simulink model "SSBaudio"  (R2015b)
settings: Solver=VariableStepAuto  StartTime=0.0  StopTime=10.0  RelTol=1e-3
undefined symbols (not defined in the file): SF_Frame, SF_PSF_SampPerSym, SF_Rsymbol
libraries: simrfV2util1 x4, dspxfrm3 x2, simrfV2elements x2, commanapbnd3 x2, commrflib2 x1, simrfV2sources1 x1, dspvision x1, commfilt2 x1
settings Model: Creator=dominikguz  LastModifiedBy=dominikguz

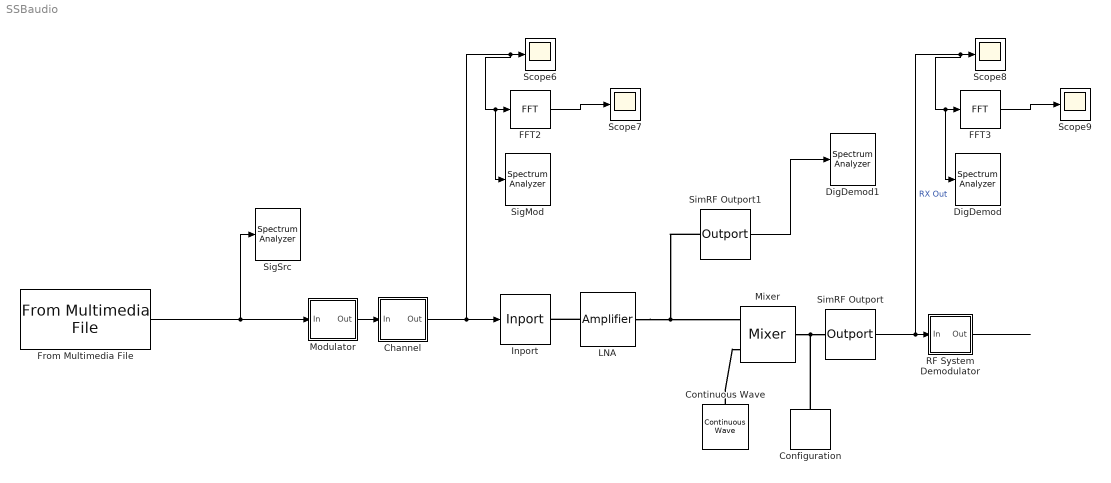
== system SSBaudio ==
  Channel : Subsystem
  Configuration : simrfV2util1/Configuration  AutoFreq=off  Tones="[5e8, 1.6e9]  Hz"  Harmonics=1  NormalizeCarrierPower=on  SolverType=Auto  StepSize=1/(SF_PSF_SampPerSym*SF_Rsymbol) s  AddNoise=on  Temperature=290.0 K  SolverDelFlag=0
  Continuous Wave : simrfV2sources1/Continuous Wave  CWSourceType=Ideal voltage  Z0=0  IVoltage=1 V  ICurrent=0 A  MagPower=0 W  QVoltage=0 V  QCurrent=0 A  AnglePower=0  CarrierFreq=SF_LO Hz  InternalGrounding=on
  DigDemod : SpectrumAnalyzer
  DigDemod1 : SpectrumAnalyzer
  FFT2 : dspxfrm3/FFT  FFTImplementation=Auto  CompMethod=Table lookup  TableOpt=NEW  TableOptActive=Speed  BitRevOrder=off  Normalize=off  InheritFFTLength=on  FFTLength=64  WrapInput=on  roundingMode=Floor  overflowMode=off  firstCoeffDataTypeStr=Inherit: Same word length as input  firstCoeffLastDataTypeStr=Inherit: Same word length as input  outputMin=[]  outputMax=[]
  FFT3 : dspxfrm3/FFT  FFTImplementation=Auto  CompMethod=Table lookup  TableOpt=NEW  TableOptActive=Speed  BitRevOrder=off  Normalize=off  InheritFFTLength=on  FFTLength=64  WrapInput=on  roundingMode=Floor  overflowMode=off  firstCoeffDataTypeStr=Inherit: Same word length as input  firstCoeffLastDataTypeStr=Inherit: Same word length as input  outputMin=[]  outputMax=[]
  From Multimedia File : dspvision/From Multimedia File  inputFilename=guitartune.wav  loop=on  numPlays=1  outputStreams=Audio only  videoDataType=single  audioDataType=double  inheritSampleTime=on  userDefinedSampleTime=1/4410  noAudioOutput=off  isIntensityVideo=off  fourcc=RGB  colorVideoFormat=Separate color signals  outputEOF=off  dataOrg=Column-major  audioFrameSize=4410  computeAudioFrameSize=off  outSamplingMode=Sample based
  Inport : simrfV2util1/Inport  SimulinkInputSignalType=Power  CarrierFreq=SF_RF Hz  ZS=50  InternalGrounding=on
  LNA : simrfV2elements/Amplifier  classname=amplifier  DataSource=Data file  File=simrfV2_unitygain.s2p  Paramtype=S-parameters  Sparam=[0 0;1 0]  SparamFreq=1e9 Hz  SparamZ0=50  Residues=0  Poles=0  DF={0 0; 1 0}  Source_linear_gain=Available power gain  linear_gain=SF_Gain_LNA dB  Zin=50  Zout=50  Source_Poly=Even and odd order  Poly_Coeffs=[0 1]  IPType=Output  IP2=inf dBm  IP3=inf dBm  P1dB=inf dBm  Psat=inf dBm  Gcomp=inf dBm  NF=SF_NoiseFigure_LNA  InternalGrounding=on  SourceFreq=Extracted from data source  PlotFreq=0 Hz  PlotType=X-Y plane  YParam1=S11  YFormat1=Magnitude (decibels)  YParam2=None  YFormat2=Magnitude (decibels)  YOption=Linear  XOption=Linear  SparamRepresentation=Time domain (rationalfit)  FitTol=-40  FitOpt=Share all poles  AutoImpulseLength=off  ImpulseLength=0 s
  Mixer : simrfV2elements/Mixer  classname=mixer  Source_linear_gain=Available power gain  linear_gain=SF_Gain_Mixer dB  Zin=50  Zout=50  ZLO=inf  Source_Poly=Even and odd order  Poly_Coeffs=0  IPType=Output  IP2=Inf dBm  IP3=Inf dBm  P1dB=Inf dBm  Psat=Inf dBm  Gcomp=Inf dBm  NF=SF_NoiseFigure_Mixer  InternalGrounding=on
  Modulator : Subsystem
  RF System Demodulator : Subsystem
  Scope{6..9} (4 alike) : Scope
  SigMod : SpectrumAnalyzer
  SigSrc : SpectrumAnalyzer
  SimRF Outport : simrfV2util1/Outport  SensorType=Power  OutputFormat=Complex Baseband  CarrierFreq="SF_IFreq  Hz"  ZL=50  InternalGrounding=on  StepSize=-1 s  AutoStep=off
  SimRF Outport1 : simrfV2util1/Outport  SensorType=Power  OutputFormat=Complex Baseband  CarrierFreq="SF_IFreq  Hz"  ZL=50  InternalGrounding=on  StepSize=-1 s  AutoStep=off
  wires:
  Modulator/1(Out) -> Channel/1(In)
  SimRF Outport/1 -> DigDemod/1, FFT3/1, Scope8/1, RF System Demodulator/1(In)  "RX Out"
  RF System Demodulator/1(Out) -> ?
  Channel/1(Out) -> SigMod/1, FFT2/1, Scope6/1, Inport/1
  FFT2/1 -> Scope7/1
  FFT3/1 -> Scope9/1
  SimRF Outport1/1 -> DigDemod1/1
  From Multimedia File/1 -> SigSrc/1, Modulator/1(In)
  connections:
  Configuration/LConn1 -- Mixer/RConn1 -- SimRF Outport/LConn1
  Continuous Wave/LConn1 -- Mixer/LConn2
  LNA/RConn1 -- SimRF Outport1/LConn1 -- Mixer/LConn1
  LNA/LConn1 -- Inport/RConn1

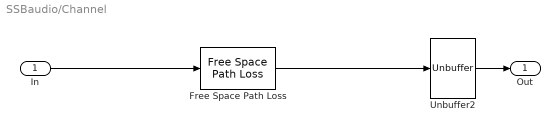
== system SSBaudio/Channel ==
  In : Inport
  Free Space Path Loss : commrflib2/Free Space Path Loss  mode=Decibels  dB=120  d=0.100  fc=1920
  Unbuffer2 : Unbuffer  SampleBasedProcessing=Same as frame based
  Out : Outport
  wires:
  Free Space Path Loss/1 -> Unbuffer2/1
  Unbuffer2/1 -> Out/1
  In/1 -> Free Space Path Loss/1

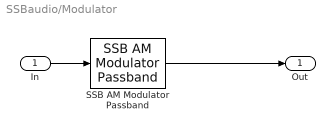
== system SSBaudio/Modulator ==
  In : Inport
  SSB AM Modulator Passband : commanapbnd3/SSB AM Modulator Passband  Fc=300  Ph=0  Sd=Upper  Ho=100
  Out : Outport
  wires:
  In/1 -> SSB AM Modulator Passband/1
  SSB AM Modulator Passband/1 -> Out/1

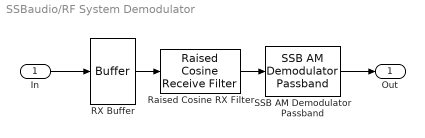
== system SSBaudio/RF System Demodulator ==
  In : Inport
  RX Buffer : Buffer  N=SF_PSF_SampPerSym*SF_Frame  TreatMby1Signals=One channel
  Raised Cosine RX Filter : commfilt2/Raised Cosine Receive Filter  filtType=Square root  N=SF_PSF_SampPerSym  filtSpan=8  currentFiltSpan=8  D=(8)/2  R=0.2  sampMode=Mute  saveAsFlag=0  rateMode=Downsampling  downFactor=SF_PSF_SampPerSym  downOffset=0  framing=Enforce single-rate processing  InputProcessing=Columns as channels (frame based)  checkGain=Normalized  filterGain=1  checkCoeff=off  variableName=rcRxFilt2  launchFVT=off  roundingMode=Floor  overflowMode=off
  SSB AM Demodulator Passband : commanapbnd3/SSB AM Demodulator Passband  Fc=300  Ph=0  method=Butterworth  n=4  cf=300  Rp=0.1  Rs=50
  Out : Outport
  wires:
  Raised Cosine RX Filter/1 -> SSB AM Demodulator Passband/1
  SSB AM Demodulator Passband/1 -> Out/1
  In/1 -> RX Buffer/1
  RX Buffer/1 -> Raised Cosine RX Filter/1
